simulink model "pid_crane"  (R2022b)
settings: Solver=VariableStepAuto  StartTime=0.0  StopTime=20  RelTol=1e-3
values from neighbouring files (symbols this model uses):
  Bc = 0.25    [parametros.m]
  Bp = 0.1    [parametros.m]
  g = 9.81    [parametros.m]    (also in pendulum_cart_control_transfer_function.m)
  Kdtheta = 7.3272e-05    [parametros.m]
  Kdx = 15    [parametros.m]
  Kitheta = 3.2605e-04    (= 0.00032605)    [parametros.m]
  Kix = 7    [parametros.m]
  Kptheta = 5.8757e-05    [parametros.m]
  Kpx = 20    [parametros.m]
  l = 0.6    [parametros.m]    (also in pendulum_cart_control_transfer_function.m)
  mc = 0.250    (= 0.25)    [parametros.m]
  mp = 0.5    [parametros.m]
settings Model: Creator=Usuario  LastModifiedBy=Carlo

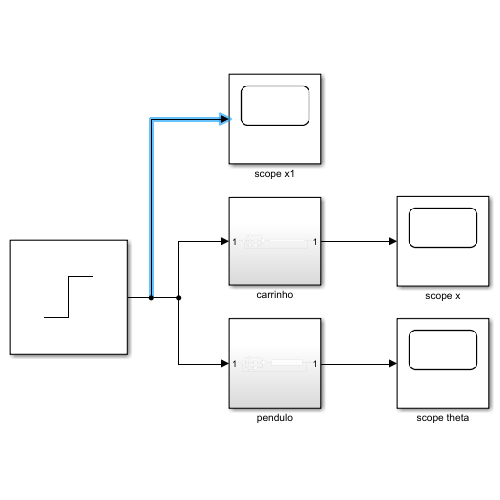
[thumbnail: Simulink's stored preview of the top-level diagram]
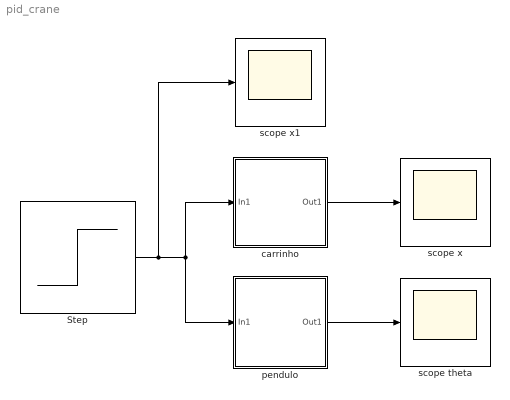
== system pid_crane ==
  Step : Step  SampleTime=0
  carrinho : Subsystem
  pendulo : Subsystem
  scope theta : Scope
  scope x : Scope
  scope x1 : Scope
  wires:
  Step/1 -> scope x1/1, pendulo/1(In1), carrinho/1(In1)
  carrinho/1(Out1) -> scope x/1
  pendulo/1(Out1) -> scope theta/1

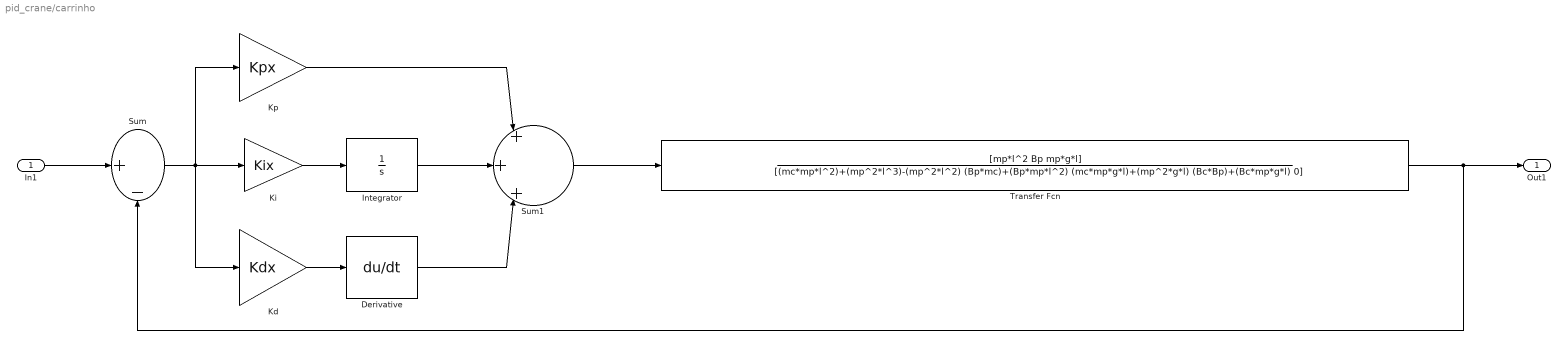
== system pid_crane/carrinho ==
  In1 : Inport
  Derivative : Derivative
  Integrator : Integrator
  Kd : Gain  Gain=Kdx
  Ki : Gain  Gain=Kix
  Kp : Gain  Gain=Kpx
  Sum : Sum  Inputs=|+-
  Sum1 : Sum  Inputs=|+|+|+|
  Transfer Fcn : TransferFcn  Numerator=[mp*l^2 Bp mp*g*l]  Denominator=[(mc*mp*l^2)+(mp^2*l^3)-(mp^2*l^2) (Bp*mc)+(Bp*mp*l^2) (mc*mp*g*l)+(mp^2*g*l) (Bc*Bp)+(Bc*mp*g*l) 0]
  Out1 : Outport
  wires:
  Transfer Fcn/1 -> Out1/1, Sum/2
  Sum/1 -> Kd/1, Kp/1, Ki/1
  Derivative/1 -> Sum1/3
  Sum1/1 -> Transfer Fcn/1
  Integrator/1 -> Sum1/2
  Kd/1 -> Derivative/1
  Ki/1 -> Integrator/1
  Kp/1 -> Sum1/1
  In1/1 -> Sum/1

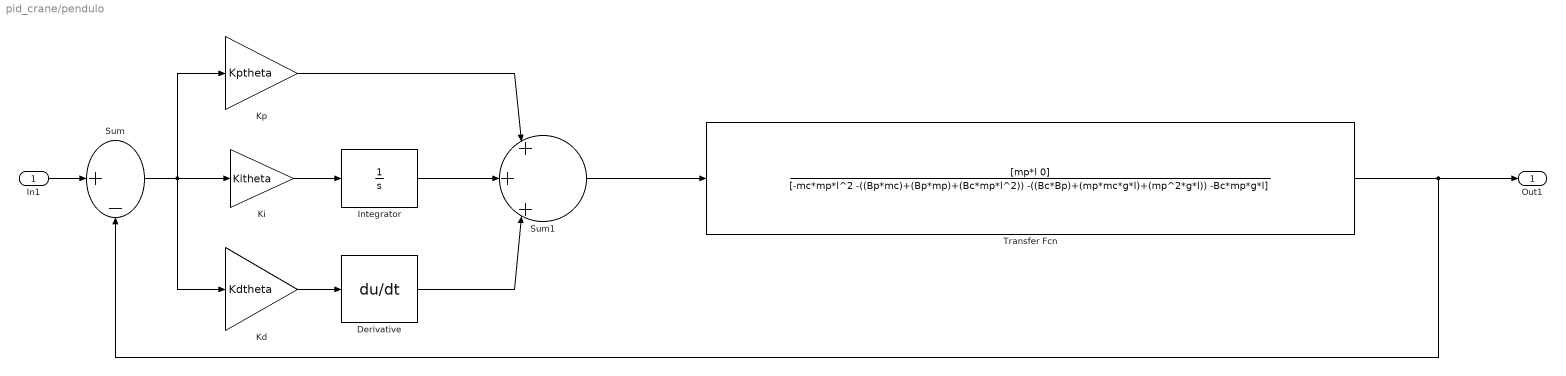
== system pid_crane/pendulo ==
  In1 : Inport
  Derivative : Derivative
  Integrator : Integrator
  Kd : Gain  Gain=Kdtheta
  Ki : Gain  Gain=Kitheta
  Kp : Gain  Gain=Kptheta
  Sum : Sum  Inputs=|+-
  Sum1 : Sum  Inputs=|+|+|+|
  Transfer Fcn : TransferFcn  Numerator=[mp*l 0]  Denominator=[-mc*mp*l^2 -((Bp*mc)+(Bp*mp)+(Bc*mp*l^2)) -((Bc*Bp)+(mp*mc*g*l)+(mp^2*g*l)) -Bc*mp*g*l]
  Out1 : Outport
  wires:
  Kd/1 -> Derivative/1
  Derivative/1 -> Sum1/3
  Kp/1 -> Sum1/1
  Sum1/1 -> Transfer Fcn/1
  Integrator/1 -> Sum1/2
  Transfer Fcn/1 -> Sum/2, Out1/1
  Ki/1 -> Integrator/1
  Sum/1 -> Kd/1, Kp/1, Ki/1
  In1/1 -> Sum/1
